simulink model "tfg"  (R2020b)
settings: Solver=VariableStepAuto  StartTime=0.0  StopTime=1  RelTol=1e-3
values from neighbouring files (symbols this model uses):
  k = 0.814    [tfgm.m]
  Kic = R/Tc    (= 500)    [tfgm.m]
  Kpc = L/Tc    (= 5.4)    [tfgm.m]
  P_ = -7000    [tfgm.m]
  Q_ = -5000    [tfgm.m]
undefined symbols (not defined in the file or in its folder): ll, rl
libraries: powerlib x11, pid_lib x2
settings Model: Creator=ssivo  LastModifiedBy=ssivo
settings SolverCC: AlgebraicLoopSolver=LineSearch

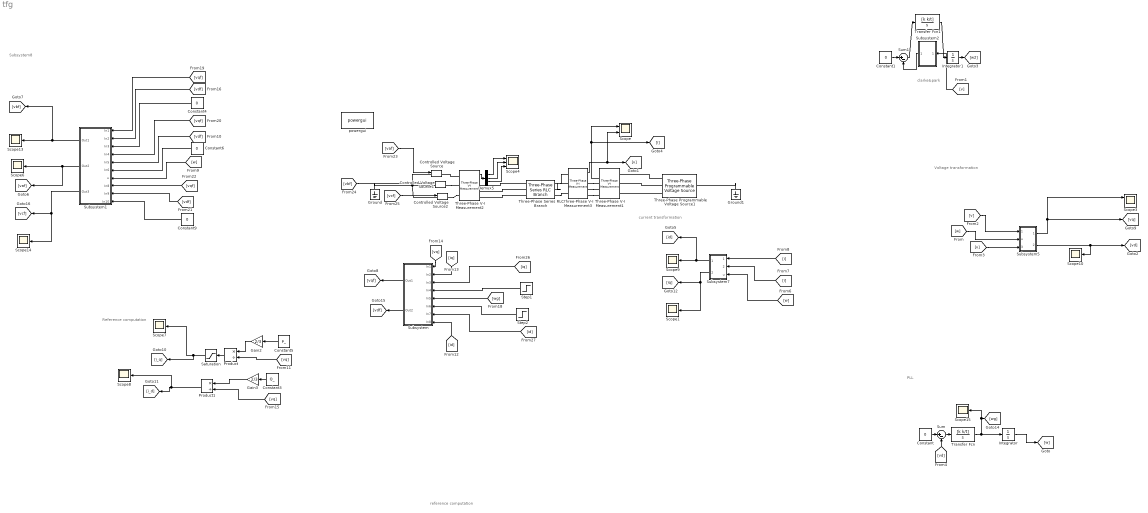
== system tfg ==
  note: Subsystem8
  note: Voltage transformation
  note: PLL
  note: current transformation
  note: Reference computation
  note: reference computation
  note: clarke&park
  Constant{,1,4,6,9} (5 alike) : Constant  Value=0
  Constant3 : Constant  Value=Q_
  Constant5 : Constant  Value=P_
  Controlled Voltage Source : powerlib/Electrical Sources/Controlled Voltage Source  Initialize=on  Source_Type=AC  Amplitude=400  Phase=0  Frequency=50  Measurements=None
  Controlled Voltage Source1 : powerlib/Electrical Sources/Controlled Voltage Source  Initialize=on  Source_Type=AC  Amplitude=400  Phase=0  Frequency=50  Measurements=None
  Controlled Voltage Source2 : powerlib/Electrical Sources/Controlled Voltage Source  Initialize=on  Source_Type=AC  Amplitude=400  Phase=0  Frequency=50  Measurements=None
  Demux5 : Demux  Outputs=3
  Gain2 : Gain  Gain=2/3
  Gain3 : Gain  Gain=2/3
  Ground : powerlib/Elements/Ground  LConnTagsString=a
  Ground1 : powerlib/Elements/Ground  LConnTagsString=a
  Integrator : Integrator
  Integrator1 : Integrator
  Product : Product  Inputs=*/
  Product1 : Product  Inputs=*/
  Saturation : Saturate  UpperLimit=0  LowerLimit=-15
  Scope : Scope  NumInputPorts=2
  Scope{1,6..10,13..15} (9 alike) : Scope
  Scope3 : Scope  NumInputPorts=2
  Scope4 : Scope  NumInputPorts=3
  Step1 : Step  Time=0.2  After=-14.29  SampleTime=0
  Step2 : Step  Time=0.1  After=-10.21  SampleTime=0
  Subsystem : Subsystem
  Subsystem1 : Subsystem
  Subsystem2 : Subsystem
  Subsystem5 : Subsystem
  Subsystem7 : Subsystem
  Sum : Sum  Inputs=|+-
  Sum1 : Sum  Inputs=|+-
  Three-Phase Programmable Voltage Source1 : powerlib/Electrical Sources/Three-Phase Programmable Voltage Source  PositiveSequence="[400  0 50]"  VariationEntity=None  VariationType=Table of time-amplitude pairs  VariationTypeAlt=Step  VariationStep=0.5  VariationRate=10  VariationMagnitude=0.3  VariationFrequency=2  VariationTiming=[1 2]  VariationPhaseA=off  Amplitudes=[1 0.8 1.2 1.0]  TimeValues=[0 0.1 0.15 0.2]  HarmonicGeneration=off  HarmonicA=[3 0.2 -25 0]  HarmonicB=[2 0.15 35 2]  Timing="[0.05  3]"  BusType=swing  Pref=0  Qref=0  Qmin=-inf  Qmax=inf
  Three-Phase Series RLC Branch : powerlib/Elements/Three-Phase Series RLC Branch  LConnTagsString=A|B|C  RConnTagsString=A|B|C  BranchType=RL  Resistance=rl  Inductance=ll  Capacitance=1e-6  Measurements=Branch currents
  Three-Phase V-I Measurement1 : powerlib/Measurements/Three-Phase V-I Measurement  VoltageMeasurement=phase-to-ground  SetLabelV=off  LabelV=Vabc  Vpu=off  VpuLL=off  CurrentMeasurement=yes  SetLabelI=off  LabelI=Iabc  Ipu=off  Pbase=100e6  Vbase=500e3  OutputType=Complex  PhasorSimulation=off  PSBequivalent=0
  Three-Phase V-I Measurement2 : powerlib/Measurements/Three-Phase V-I Measurement  VoltageMeasurement=phase-to-ground  SetLabelV=off  LabelV=Vabc  Vpu=off  VpuLL=off  CurrentMeasurement=yes  SetLabelI=off  LabelI=Iabc  Ipu=off  Pbase=100e6  Vbase=500e3  OutputType=Complex  PhasorSimulation=off  PSBequivalent=0
  Three-Phase V-I Measurement3 : powerlib/Measurements/Three-Phase V-I Measurement  VoltageMeasurement=phase-to-ground  SetLabelV=off  LabelV=Vabc  Vpu=off  VpuLL=off  CurrentMeasurement=yes  SetLabelI=off  LabelI=Iabc  Ipu=off  Pbase=100e6  Vbase=500e3  OutputType=Complex  PhasorSimulation=off  PSBequivalent=0
  Transfer Fcn : TransferFcn  Numerator=[k k/t]  Denominator=[1 0]
  Transfer Fcn1 : TransferFcn  Numerator=[k k/t]  Denominator=[1 0]
  powergui : powerlib/powergui  Priority=1  SimulationMode=Continuous  SampleTime=1e-5  frequency=60  Iterations=50  frequencyindice=50  Pbase=100e6  ErrMax=1e-4  UnitsV=kV  UnitsW=MW  buscounter=0  FunctionMessages=off  echomessages=off  EnableUseOfTLC=off  CurrentSourceSwitches=off  DisableSnubberDevices=off  DisableRonSwitches=off  DisableVfSwitches=off  DisplayEquations=off  AutomaticDiscreteSolvers=off  SolverType=Tustin/Backward Euler (TBE)  Interpol=off  ExternalGateDelay=off  methode=off  Ts=100  x0status=blocks  SPID=on  SwTol=0  HookPort=off  NonlinearTolerance=1e-4  nMaxIteration=100  ContinueOnMaxIteration=off  RestoreLinks=warning  ResistiveCurrentMeasurement=off  Frange=[0:2:500]  Ylog=off  Xlog=on  ShowGrid=off  save=off  variable=ZData  structure=0  ZoomFFT=off  StartTime=0.0  cycles=1  DisplayStyle=1  fundamental=60  FreqAxis=off  MaxFrequency=1000  frequencyindicesteady=1  RmsSteady=1  display=off
  wires:
  Transfer Fcn/1 -> Scope15/1, [wg], Integrator/1
  Constant/1 -> Sum/1
  Sum/1 -> Transfer Fcn/1
  [vd] -> Sum/2
  Sum1/1 -> Transfer Fcn1/1
  Transfer Fcn1/1 -> Integrator1/1
  Constant1/1 -> Sum1/1
  Integrator1/1 -> [w2]
  Subsystem2/1(Out1) -> Sum1/2
  [v] -> Subsystem2/1(In1)
  Three-Phase V-I Measurement1/2 -> [i], Scope/1
  Three-Phase V-I Measurement2/1 -> Demux5/1
  Demux5/1 -> Scope4/1
  Gain3/1 -> Product1/1
  Constant3/1 -> Gain3/1
  [vq] -> Product1/2
  Constant5/1 -> Gain2/1
  [vq] -> Product/2
  Gain2/1 -> Product/1
  Product/1 -> Saturation/1
  Product1/1 -> Scope8/1, [i_d]
  Demux5/2 -> Scope4/2
  Demux5/3 -> Scope4/3
  Integrator/1 -> [w]
  [vaf] -> Controlled Voltage Source/1
  [vbf] -> Controlled Voltage Source1/1
  [vcf] -> Controlled Voltage Source2/1
  Saturation/1 -> [i_q], Scope7/1
  [vq] -> Subsystem/1(In1)
  [iq] -> Subsystem/2(In2)
  [iq] -> Subsystem/3(In3)
  Step1/1 -> Subsystem/4(In4)
  [wg] -> Subsystem/5(In5)
  Step2/1 -> Subsystem/6(In6)
  [id] -> Subsystem/7(In7)
  [id] -> Subsystem/8(In8)
  Subsystem/1(Out1) -> [vqf]
  Subsystem/2(Out2) -> [vdf]
  Subsystem1/2(Out2) -> Scope6/1, [vaf]
  Subsystem1/3(Out3) -> Scope14/1, [vcf]
  Subsystem1/1(Out1) -> [vbf], Scope13/1
  [vqf] -> Subsystem1/1(In1)
  [vdf] -> Subsystem1/2(In2)
  Constant4/1 -> Subsystem1/3(In3)
  [vqf] -> Subsystem1/4(In4)
  [vdf] -> Subsystem1/5(In5)
  Constant6/1 -> Subsystem1/6(In6)
  [w] -> Subsystem1/7(u)
  [vqf] -> Subsystem1/8(In8)
  [vdf] -> Subsystem1/9(In9)
  Constant9/1 -> Subsystem1/10(In10)
  Subsystem7/2(Out2) -> Scope1/1, [iq]
  Subsystem7/1(Out1) -> [id], Scope9/1
  [i] -> Subsystem7/1(In1)
  [i] -> Subsystem7/2(In2)
  [w] -> Subsystem7/3(u)
  Subsystem5/2(Out2) -> Scope10/1, [vd]
  Subsystem5/1(Out1) -> Scope3/1, [vq]
  [v] -> Subsystem5/1(In1)
  [w] -> Subsystem5/2(u)
  [v] -> Subsystem5/3(In3)
  Three-Phase V-I Measurement3/1 -> Scope/2, [v]
  connections:
  Controlled Voltage Source1/RConn1 -- Three-Phase V-I Measurement2/LConn2
  Ground/LConn1 -- Controlled Voltage Source/LConn1 -- Controlled Voltage Source2/LConn1 -- Controlled Voltage Source1/LConn1
  Three-Phase V-I Measurement2/LConn1 -- Controlled Voltage Source/RConn1
  Controlled Voltage Source2/RConn1 -- Three-Phase V-I Measurement2/LConn3
  Three-Phase Programmable Voltage Source1/RConn1 -- Three-Phase V-I Measurement1/LConn1
  Three-Phase Programmable Voltage Source1/RConn2 -- Three-Phase V-I Measurement1/LConn2
  Three-Phase Programmable Voltage Source1/RConn3 -- Three-Phase V-I Measurement1/LConn3
  Ground1/LConn1 -- Three-Phase Programmable Voltage Source1/LConn1
  Three-Phase Series RLC Branch/LConn3 -- Three-Phase V-I Measurement2/RConn3
  Three-Phase Series RLC Branch/LConn2 -- Three-Phase V-I Measurement2/RConn2
  Three-Phase Series RLC Branch/LConn1 -- Three-Phase V-I Measurement2/RConn1
  Three-Phase Series RLC Branch/RConn1 -- Three-Phase V-I Measurement3/LConn1
  Three-Phase Series RLC Branch/RConn2 -- Three-Phase V-I Measurement3/LConn2
  Three-Phase Series RLC Branch/RConn3 -- Three-Phase V-I Measurement3/LConn3
  Three-Phase V-I Measurement3/RConn1 -- Three-Phase V-I Measurement1/RConn1
  Three-Phase V-I Measurement3/RConn2 -- Three-Phase V-I Measurement1/RConn2
  Three-Phase V-I Measurement3/RConn3 -- Three-Phase V-I Measurement1/RConn3

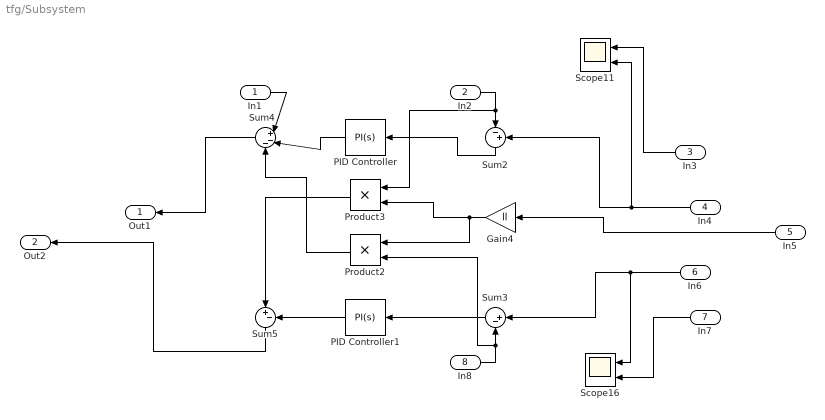
== system tfg/Subsystem ==
  In1 : Inport
  In2 : Inport  Port=2
  In3 : Inport  Port=3
  In4 : Inport  Port=4
  In5 : Inport  Port=5
  In6 : Inport  Port=6
  In7 : Inport  Port=7
  In8 : Inport  Port=8
  Gain4 : Gain  Gain=ll
  PID Controller : pid_lib/PID Controller  Controller=PI  Form=Parallel  TimeDomain=Continuous-time  UseExternalTs=off  SampleTime=-1  IntegratorMethod=Forward Euler  FilterMethod=Forward Euler  ControllerParametersSource=internal  P=Kpc  I=Kic  D=0  UseFilter=on  N=100  TunerSelectOption=Transfer Function Based (PID Tuner App)  InitialConditionSource=internal  InitialConditionForIntegrator=0  InitialConditionForFilter=0  DifferentiatorICPrevScaledInput=0  ExternalReset=none  TrackingMode=off  Kt=1  LimitOutput=off  SatLimitsSource=internal  UpperSaturationLimit=inf  LowerSaturationLimit=-inf  LinearizeAsGain=on  AntiWindupMode=none  Kb=1  POutMin=[]  POutMax=[]  IOutMin=[]  IOutMax=[]  DOutMin=[]  DOutMax=[]  NOutMin=[]  NOutMax=[]  SumOutMin=[]  SumOutMax=[]  SaturationOutMin=[]  SaturationOutMax=[]  PParamMin=[]  PParamMax=[]  IParamMin=[]  IParamMax=[]  DParamMin=[]  DParamMax=[]  NParamMin=[]  NParamMax=[]  KbParamMin=[]  KbParamMax=[]  KtParamMin=[]  KtParamMax=[]  KbOutMin=[]  KbOutMax=[]  KtOutMin=[]  KtOutMax=[]  IntegratorOutMin=[]  IntegratorOutMax=[]  FilterOutMin=[]  FilterOutMax=[]  SumI1OutMin=[]  SumI1OutMax=[]  SumI2OutMin=[]  SumI2OutMax=[]  SumI3OutMin=[]  SumI3OutMax=[]  SumI4OutMin=[]  SumI4OutMax=[]  SumDOutMin=[]  SumDOutMax=[]  DifferentiatorOutMin=[]  DifferentiatorOutMax=[]  FilterDiffOutCoefMin=[]  FilterDiffOutCoefMax=[]  ReciprocalOutMin=[]  ReciprocalOutMax=[]  SumDenOutMin=[]  SumDenOutMax=[]  SumNumOutMin=[]  SumNumOutMax=[]  DivideOutMin=[]  DivideOutMax=[]  UdiffTsProdOutMin=[]  UdiffTsProdOutMax=[]  NTsProdOutMin=[]  NTsProdOutMax=[]  UintegralTsProdOutMin=[]  UintegralTsProdOutMax=[]  UngainTsProdOutMin=[]  UngainTsProdOutMax=[]  IntegratorContinuousStateAttributes=''  IntegratorStateMustResolveToSignalObject=off  IntegratorRTWStateStorageClass=Auto  FilterContinuousStateAttributes=''  FilterStateMustResolveToSignalObject=off  FilterRTWStateStorageClass=Auto  ParallelPVariant=InternalParameters  IdealPVariant=Disabled  IVariant=InternalParameters  DVariant=Disabled  IntegratorVariant=Continuous  SatVariant=Disabled  AWVariant=Passthrough  PCopyVariant=Disabled  TRVariant=Disabled  FdbkBlocksVariant=Forward  IdealPFdbkVariant=Disabled  SatFdbkVariant=Disabled  DerivativeFilterVariant=Disabled  NVariant=Disabled  NCopyVariant=Disabled_SignalSpec  FilterICVariant=Disabled  IntegratorICVariant=InternalICs  ExternalResetVariant=Disabled  TRSumVariant=Passthrough  SumFdbkVariant=Disabled  SumVariant=Sum_PI  TsampFilterVariant=InternalTs  TsampNgainVariant=Passthrough  TsampIntegralVariant=Passthrough  ExternalSaturationOutDataTypeStr=Inherit: Same as second input
  PID Controller1 : pid_lib/PID Controller  Controller=PI  Form=Parallel  TimeDomain=Continuous-time  UseExternalTs=off  SampleTime=-1  IntegratorMethod=Forward Euler  FilterMethod=Forward Euler  ControllerParametersSource=internal  P=Kpc  I=Kic  D=0  UseFilter=on  N=100  TunerSelectOption=Transfer Function Based (PID Tuner App)  InitialConditionSource=internal  InitialConditionForIntegrator=0  InitialConditionForFilter=0  DifferentiatorICPrevScaledInput=0  ExternalReset=none  TrackingMode=off  Kt=1  LimitOutput=off  SatLimitsSource=internal  UpperSaturationLimit=inf  LowerSaturationLimit=-inf  LinearizeAsGain=on  AntiWindupMode=none  Kb=1  POutMin=[]  POutMax=[]  IOutMin=[]  IOutMax=[]  DOutMin=[]  DOutMax=[]  NOutMin=[]  NOutMax=[]  SumOutMin=[]  SumOutMax=[]  SaturationOutMin=[]  SaturationOutMax=[]  PParamMin=[]  PParamMax=[]  IParamMin=[]  IParamMax=[]  DParamMin=[]  DParamMax=[]  NParamMin=[]  NParamMax=[]  KbParamMin=[]  KbParamMax=[]  KtParamMin=[]  KtParamMax=[]  KbOutMin=[]  KbOutMax=[]  KtOutMin=[]  KtOutMax=[]  IntegratorOutMin=[]  IntegratorOutMax=[]  FilterOutMin=[]  FilterOutMax=[]  SumI1OutMin=[]  SumI1OutMax=[]  SumI2OutMin=[]  SumI2OutMax=[]  SumI3OutMin=[]  SumI3OutMax=[]  SumI4OutMin=[]  SumI4OutMax=[]  SumDOutMin=[]  SumDOutMax=[]  DifferentiatorOutMin=[]  DifferentiatorOutMax=[]  FilterDiffOutCoefMin=[]  FilterDiffOutCoefMax=[]  ReciprocalOutMin=[]  ReciprocalOutMax=[]  SumDenOutMin=[]  SumDenOutMax=[]  SumNumOutMin=[]  SumNumOutMax=[]  DivideOutMin=[]  DivideOutMax=[]  UdiffTsProdOutMin=[]  UdiffTsProdOutMax=[]  NTsProdOutMin=[]  NTsProdOutMax=[]  UintegralTsProdOutMin=[]  UintegralTsProdOutMax=[]  UngainTsProdOutMin=[]  UngainTsProdOutMax=[]  IntegratorContinuousStateAttributes=''  IntegratorStateMustResolveToSignalObject=off  IntegratorRTWStateStorageClass=Auto  FilterContinuousStateAttributes=''  FilterStateMustResolveToSignalObject=off  FilterRTWStateStorageClass=Auto  ParallelPVariant=InternalParameters  IdealPVariant=Disabled  IVariant=InternalParameters  DVariant=Disabled  IntegratorVariant=Continuous  SatVariant=Disabled  AWVariant=Passthrough  PCopyVariant=Disabled  TRVariant=Disabled  FdbkBlocksVariant=Forward  IdealPFdbkVariant=Disabled  SatFdbkVariant=Disabled  DerivativeFilterVariant=Disabled  NVariant=Disabled  NCopyVariant=Disabled_SignalSpec  FilterICVariant=Disabled  IntegratorICVariant=InternalICs  ExternalResetVariant=Disabled  TRSumVariant=Passthrough  SumFdbkVariant=Disabled  SumVariant=Sum_PI  TsampFilterVariant=InternalTs  TsampNgainVariant=Passthrough  TsampIntegralVariant=Passthrough  ExternalSaturationOutDataTypeStr=Inherit: Same as second input
  Product2 : Product
  Product3 : Product
  Scope11 : Scope  NumInputPorts=2
  Scope16 : Scope  NumInputPorts=2
  Sum2 : Sum  Inputs=|-+
  Sum3 : Sum  Inputs=|+-
  Sum4 : Sum  Inputs=|+--
  Sum5 : Sum  Inputs=|+-
  Out1 : Outport
  Out2 : Outport  Port=2
  wires:
  Sum2/1 -> PID Controller/1
  In4/1 -> Sum2/2, Scope11/2
  Sum3/1 -> PID Controller1/1
  In6/1 -> Sum3/1, Scope16/1
  PID Controller/1 -> Sum4/2
  Product3/1 -> Sum5/1
  In1/1 -> Sum4/1
  In2/1 -> Product3/1, Sum2/1
  In3/1 -> Scope11/1
  Product2/1 -> Sum4/3
  In8/1 -> Product2/2, Sum3/2
  Gain4/1 -> Product2/1, Product3/2
  PID Controller1/1 -> Sum5/2
  In7/1 -> Scope16/2
  Sum5/1 -> Out2/1
  Sum4/1 -> Out1/1
  In5/1 -> Gain4/1

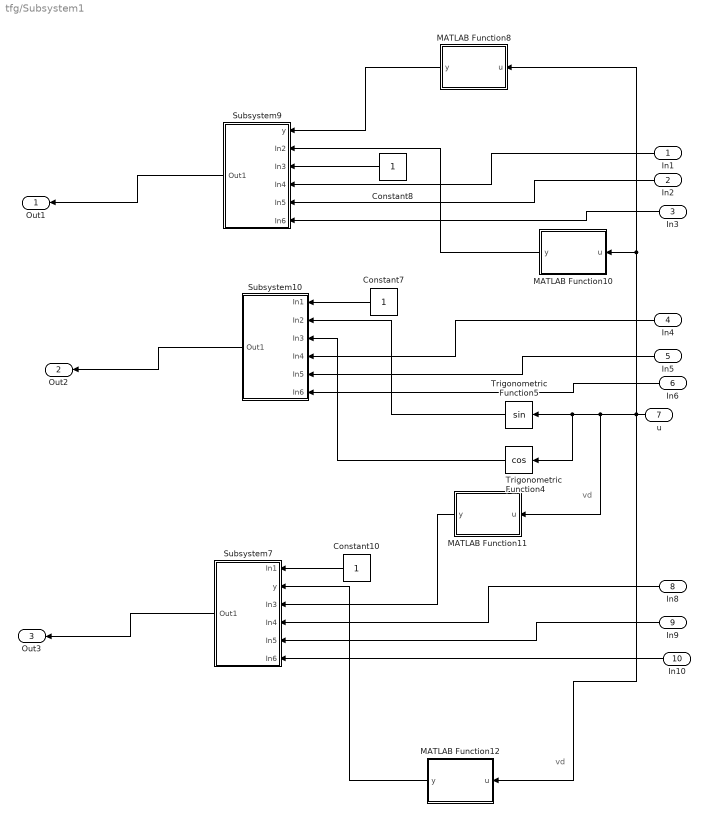
== system tfg/Subsystem1 ==
  note: vd
  note: vd
  In1 : Inport
  In2 : Inport  Port=2
  In3 : Inport  Port=3
  In4 : Inport  Port=4
  In5 : Inport  Port=5
  In6 : Inport  Port=6
  u : Inport  Port=7
  In8 : Inport  Port=8
  In9 : Inport  Port=9
  In10 : Inport  Port=10
  Constant10 : Constant
  Constant7 : Constant
  Constant8 : Constant
  MATLAB Function10 : MATLAB Function  TreatAsAtomicUnit=on
  MATLAB Function11 : MATLAB Function  TreatAsAtomicUnit=on
  MATLAB Function12 : MATLAB Function  TreatAsAtomicUnit=on
  MATLAB Function8 : MATLAB Function  TreatAsAtomicUnit=on
  Subsystem10 : Subsystem
  Subsystem7 : Subsystem
  Subsystem9 : Subsystem
  Trigonometric Function4 : Trigonometry  Operator=cos
  Trigonometric Function5 : Trigonometry
  Out1 : Outport
  Out2 : Outport  Port=2
  Out3 : Outport  Port=3
  wires:
  Trigonometric Function5/1 -> Subsystem10/2(In2)
  MATLAB Function12/1(y) -> Subsystem7/2(y)
  Trigonometric Function4/1 -> Subsystem10/3(In3)
  u/1 -> MATLAB Function12/1(u), MATLAB Function11/1(u), Trigonometric Function4/1, Trigonometric Function5/1, MATLAB Function10/1(u), MATLAB Function8/1(u)
  Subsystem10/1(Out1) -> Out2/1
  Constant10/1 -> Subsystem7/1(In1)
  MATLAB Function8/1(y) -> Subsystem9/1(y)
  Constant8/1 -> Subsystem9/3(In3)
  MATLAB Function11/1(y) -> Subsystem7/3(In3)
  In10/1 -> Subsystem7/6(In6)
  Subsystem7/1(Out1) -> Out3/1
  In8/1 -> Subsystem7/4(In4)
  MATLAB Function10/1(y) -> Subsystem9/2(In2)
  Constant7/1 -> Subsystem10/1(In1)
  In3/1 -> Subsystem9/6(In6)
  In4/1 -> Subsystem10/4(In4)
  In2/1 -> Subsystem9/5(In5)
  In1/1 -> Subsystem9/4(In4)
  In6/1 -> Subsystem10/6(In6)
  In5/1 -> Subsystem10/5(In5)
  In9/1 -> Subsystem7/5(In5)
  Subsystem9/1(Out1) -> Out1/1

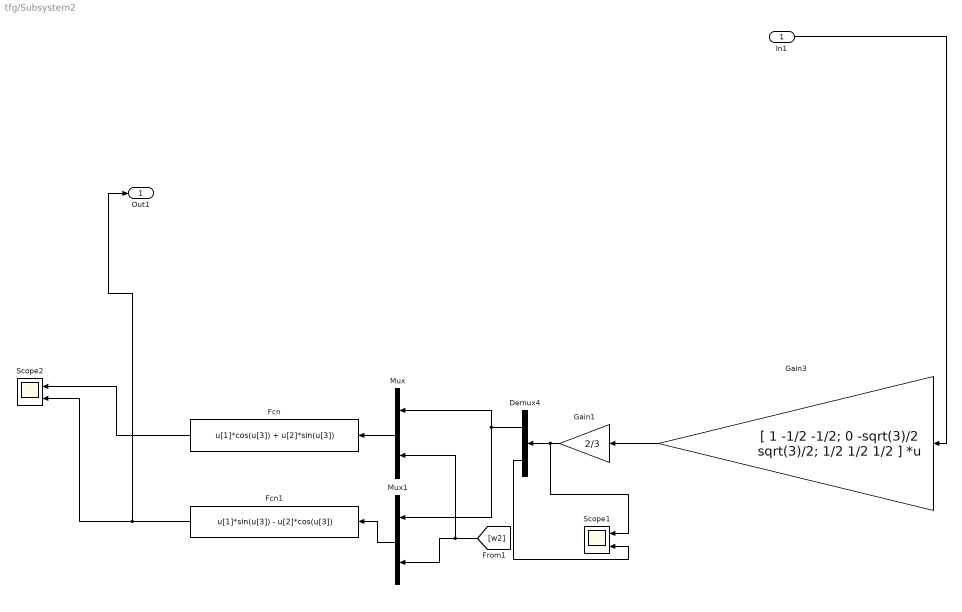
== system tfg/Subsystem2 ==
  In1 : Inport
  Demux4 : Demux  Outputs=[2 1]
  Fcn : Fcn  Expr=u[1]*cos(u[3]) + u[2]*sin(u[3])
  Fcn1 : Fcn  Expr=u[1]*sin(u[3]) - u[2]*cos(u[3])
  Gain1 : Gain  Gain=2/3  SaturateOnIntegerOverflow=on  OutDataTypeStr=Inherit: Same as input  ParamDataTypeStr=Inherit: Same as input
  Gain3 : Gain  Gain="[ 1   -1/2   -1/2; 0   -sqrt(3)/2   sqrt(3)/2; 1/2  1/2  1/2 ]"  Multiplication=Matrix(K*u) (u vector)  SaturateOnIntegerOverflow=on  OutDataTypeStr=Inherit: Same as input  ParamDataTypeStr=Inherit: Same as input
  Mux : Mux  Inputs=2
  Mux1 : Mux  Inputs=2
  Scope1 : Scope  NumInputPorts=2
  Scope2 : Scope  NumInputPorts=2
  Out1 : Outport
  wires:
  Demux4/2 -> Scope1/2
  Fcn/1 -> Scope2/1
  [w2] -> Mux/2, Mux1/2
  Gain3/1 -> Gain1/1
  Mux1/1 -> Fcn1/1
  Gain1/1 -> Scope1/1, Demux4/1
  Mux/1 -> Fcn/1
  Demux4/1 -> Mux1/1, Mux/1
  Fcn1/1 -> Out1/1, Scope2/2
  In1/1 -> Gain3/1

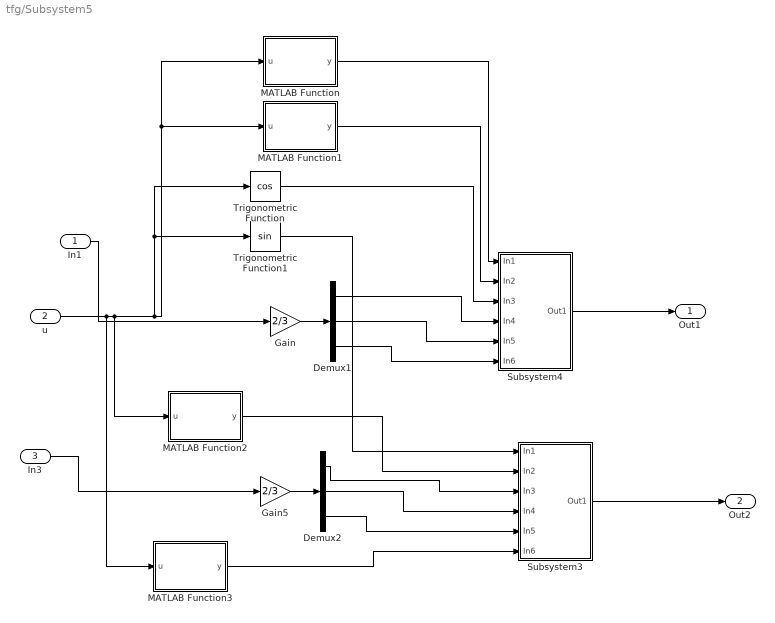
== system tfg/Subsystem5 ==
  In1 : Inport
  u : Inport  Port=2
  In3 : Inport  Port=3
  Demux1 : Demux  Outputs=[1 1 1]
  Demux2 : Demux  Outputs=[1 1 1]
  Gain : Gain  Gain=2/3
  Gain5 : Gain  Gain=2/3
  MATLAB Function : MATLAB Function  TreatAsAtomicUnit=on
  MATLAB Function1 : MATLAB Function  TreatAsAtomicUnit=on
  MATLAB Function2 : MATLAB Function  TreatAsAtomicUnit=on
  MATLAB Function3 : MATLAB Function  TreatAsAtomicUnit=on
  Subsystem3 : Subsystem
  Subsystem4 : Subsystem
  Trigonometric Function : Trigonometry  Operator=cos
  Trigonometric Function1 : Trigonometry
  Out1 : Outport
  Out2 : Outport  Port=2
  wires:
  Trigonometric Function1/1 -> Subsystem3/1(In1)
  Demux1/1 -> Subsystem4/4(In4)
  MATLAB Function3/1(y) -> Subsystem3/6(In6)
  MATLAB Function2/1(y) -> Subsystem3/2(In2)
  Demux1/3 -> Subsystem4/6(In6)
  Demux2/3 -> Subsystem3/5(In5)
  MATLAB Function/1(y) -> Subsystem4/1(In1)
  Demux2/2 -> Subsystem3/4(In4)
  Demux1/2 -> Subsystem4/5(In5)
  Demux2/1 -> Subsystem3/3(In3)
  MATLAB Function1/1(y) -> Subsystem4/2(In2)
  Trigonometric Function/1 -> Subsystem4/3(In3)
  u/1 -> MATLAB Function/1(u), MATLAB Function1/1(u), Trigonometric Function/1, Trigonometric Function1/1, MATLAB Function2/1(u), MATLAB Function3/1(u)
  Subsystem3/1(Out1) -> Out2/1
  Gain5/1 -> Demux2/1
  Gain/1 -> Demux1/1
  In3/1 -> Gain5/1
  In1/1 -> Gain/1
  Subsystem4/1(Out1) -> Out1/1

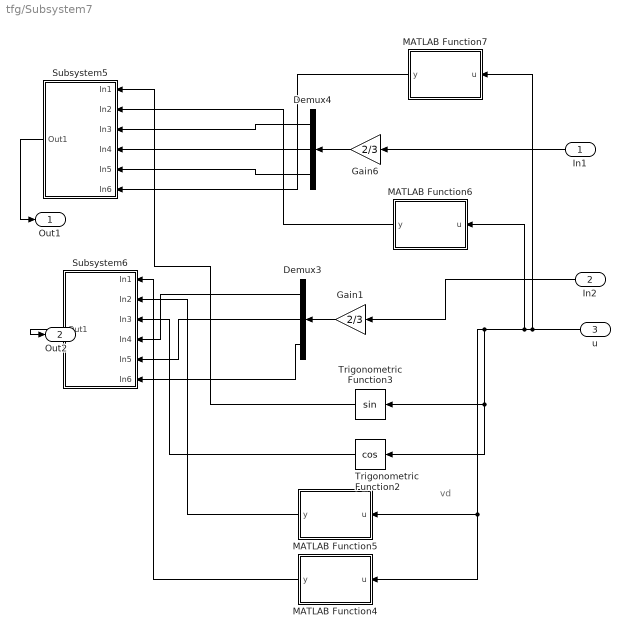
== system tfg/Subsystem7 ==
  note: vd
  In1 : Inport
  In2 : Inport  Port=2
  u : Inport  Port=3
  Demux3 : Demux  Outputs=[1 1 1]
  Demux4 : Demux  Outputs=[1 1 1]
  Gain1 : Gain  Gain=2/3
  Gain6 : Gain  Gain=2/3
  MATLAB Function4 : MATLAB Function  TreatAsAtomicUnit=on
  MATLAB Function5 : MATLAB Function  TreatAsAtomicUnit=on
  MATLAB Function6 : MATLAB Function  TreatAsAtomicUnit=on
  MATLAB Function7 : MATLAB Function  TreatAsAtomicUnit=on
  Subsystem5 : Subsystem
  Subsystem6 : Subsystem
  Trigonometric Function2 : Trigonometry  Operator=cos
  Trigonometric Function3 : Trigonometry
  Out1 : Outport
  Out2 : Outport  Port=2
  wires:
  Demux3/2 -> Subsystem6/5(In5)
  Demux3/1 -> Subsystem6/4(In4)
  Subsystem6/1(Out1) -> Out2/1
  Demux3/3 -> Subsystem6/6(In6)
  Gain1/1 -> Demux3/1
  Gain6/1 -> Demux4/1
  Demux4/3 -> Subsystem5/5(In5)
  MATLAB Function4/1(y) -> Subsystem6/1(In1)
  Trigonometric Function3/1 -> Subsystem5/1(In1)
  Trigonometric Function2/1 -> Subsystem6/3(In3)
  Demux4/1 -> Subsystem5/3(In3)
  MATLAB Function5/1(y) -> Subsystem6/2(In2)
  u/1 -> Trigonometric Function2/1, Trigonometric Function3/1, MATLAB Function5/1(u), MATLAB Function4/1(u), MATLAB Function6/1(u), MATLAB Function7/1(u)
  Demux4/2 -> Subsystem5/4(In4)
  MATLAB Function7/1(y) -> Subsystem5/6(In6)
  MATLAB Function6/1(y) -> Subsystem5/2(In2)
  In2/1 -> Gain1/1
  In1/1 -> Gain6/1
  Subsystem5/1(Out1) -> Out1/1

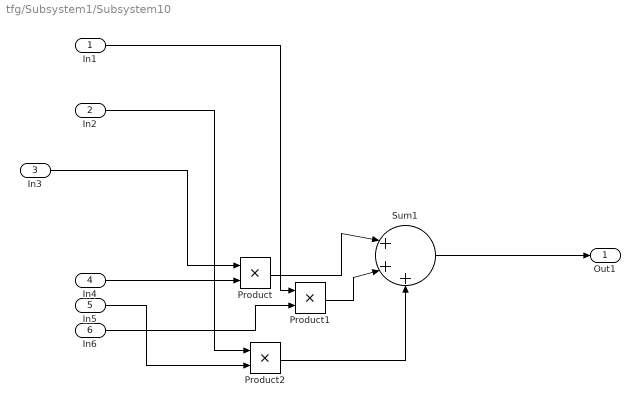
== system tfg/Subsystem1/Subsystem10 ==
  In1 : Inport
  In2 : Inport  Port=2
  In3 : Inport  Port=3
  In4 : Inport  Port=4
  In5 : Inport  Port=5
  In6 : Inport  Port=6
  Product : Product
  Product1 : Product
  Product2 : Product
  Sum1 : Sum  Inputs=|+++
  Out1 : Outport
  wires:
  Product1/1 -> Sum1/2
  In2/1 -> Product2/1
  Product2/1 -> Sum1/3
  In3/1 -> Product/1
  In5/1 -> Product2/2
  Product/1 -> Sum1/1
  In6/1 -> Product1/2
  In1/1 -> Product1/1
  In4/1 -> Product/2
  Sum1/1 -> Out1/1

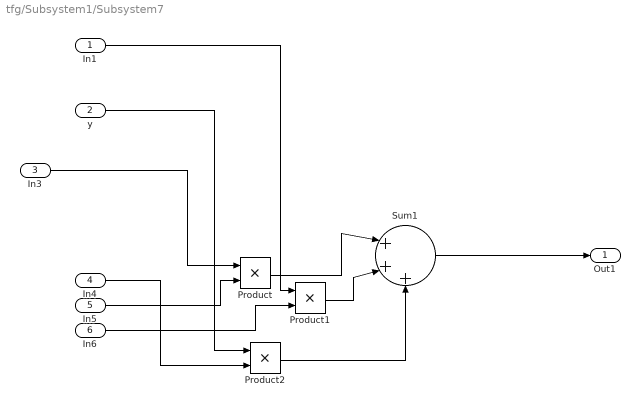
== system tfg/Subsystem1/Subsystem7 ==
  In1 : Inport
  y : Inport  Port=2
  In3 : Inport  Port=3
  In4 : Inport  Port=4
  In5 : Inport  Port=5
  In6 : Inport  Port=6
  Product : Product
  Product1 : Product
  Product2 : Product
  Sum1 : Sum  Inputs=|+++
  Out1 : Outport
  wires:
  Product1/1 -> Sum1/2
  y/1 -> Product2/1
  Product2/1 -> Sum1/3
  In3/1 -> Product/1
  In5/1 -> Product/2
  Product/1 -> Sum1/1
  In6/1 -> Product1/2
  In1/1 -> Product1/1
  In4/1 -> Product2/2
  Sum1/1 -> Out1/1

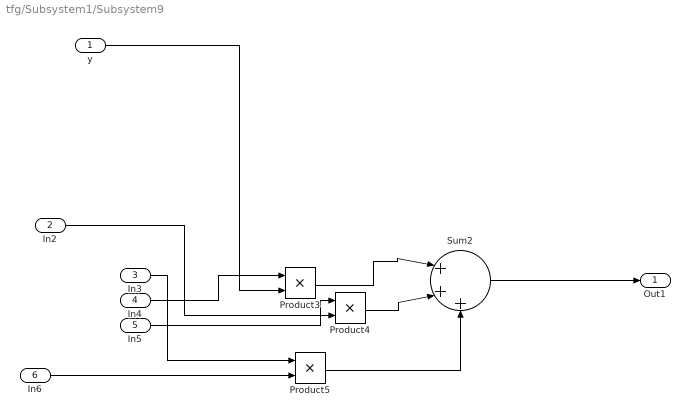
== system tfg/Subsystem1/Subsystem9 ==
  y : Inport
  In2 : Inport  Port=2
  In3 : Inport  Port=3
  In4 : Inport  Port=4
  In5 : Inport  Port=5
  In6 : Inport  Port=6
  Product3 : Product
  Product4 : Product
  Product5 : Product
  Sum2 : Sum  Inputs=|+++
  Out1 : Outport
  wires:
  In4/1 -> Product3/1
  In6/1 -> Product5/2
  Product3/1 -> Sum2/1
  Product4/1 -> Sum2/2
  In5/1 -> Product4/1
  Product5/1 -> Sum2/3
  In3/1 -> Product5/1
  y/1 -> Product3/2
  In2/1 -> Product4/2
  Sum2/1 -> Out1/1

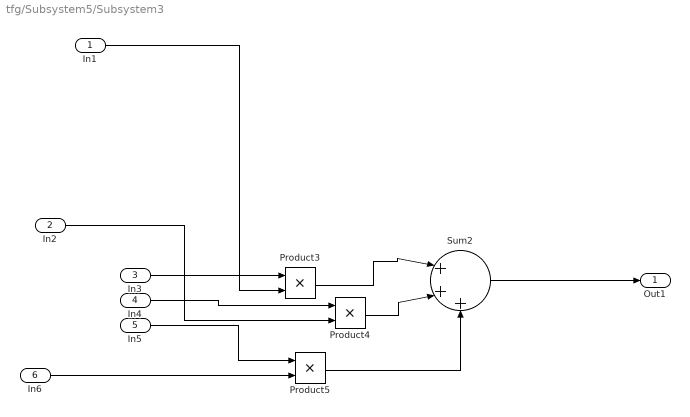
== system tfg/Subsystem5/Subsystem3 ==
  In1 : Inport
  In2 : Inport  Port=2
  In3 : Inport  Port=3
  In4 : Inport  Port=4
  In5 : Inport  Port=5
  In6 : Inport  Port=6
  Product3 : Product
  Product4 : Product
  Product5 : Product
  Sum2 : Sum  Inputs=|+++
  Out1 : Outport
  wires:
  In4/1 -> Product4/1
  In6/1 -> Product5/2
  Product3/1 -> Sum2/1
  Product4/1 -> Sum2/2
  In5/1 -> Product5/1
  Product5/1 -> Sum2/3
  In3/1 -> Product3/1
  In1/1 -> Product3/2
  In2/1 -> Product4/2
  Sum2/1 -> Out1/1

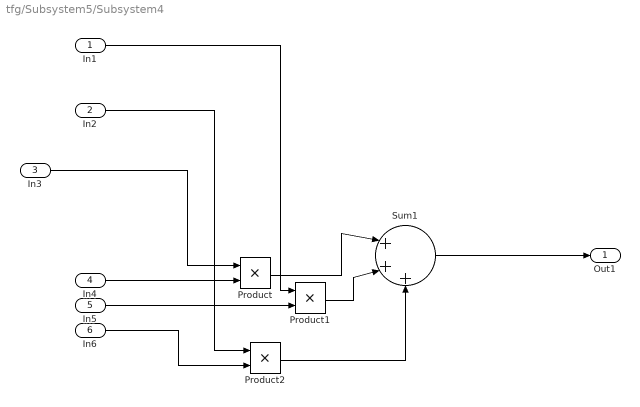
== system tfg/Subsystem5/Subsystem4 ==
  In1 : Inport
  In2 : Inport  Port=2
  In3 : Inport  Port=3
  In4 : Inport  Port=4
  In5 : Inport  Port=5
  In6 : Inport  Port=6
  Product : Product
  Product1 : Product
  Product2 : Product
  Sum1 : Sum  Inputs=|+++
  Out1 : Outport
  wires:
  Product1/1 -> Sum1/2
  In2/1 -> Product2/1
  Product2/1 -> Sum1/3
  In3/1 -> Product/1
  In5/1 -> Product1/2
  Product/1 -> Sum1/1
  In6/1 -> Product2/2
  In1/1 -> Product1/1
  In4/1 -> Product/2
  Sum1/1 -> Out1/1

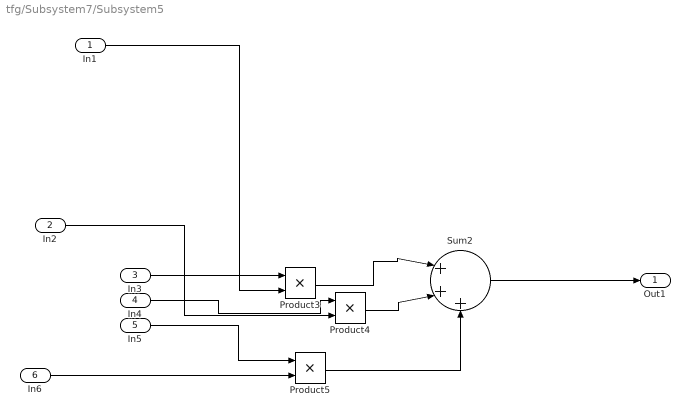
== system tfg/Subsystem7/Subsystem5 ==
  In1 : Inport
  In2 : Inport  Port=2
  In3 : Inport  Port=3
  In4 : Inport  Port=4
  In5 : Inport  Port=5
  In6 : Inport  Port=6
  Product3 : Product
  Product4 : Product
  Product5 : Product
  Sum2 : Sum  Inputs=|+++
  Out1 : Outport
  wires:
  In4/1 -> Product4/1
  In6/1 -> Product5/2
  Product3/1 -> Sum2/1
  Product4/1 -> Sum2/2
  In5/1 -> Product5/1
  Product5/1 -> Sum2/3
  In3/1 -> Product3/1
  In1/1 -> Product3/2
  In2/1 -> Product4/2
  Sum2/1 -> Out1/1

== system tfg/Subsystem7/Subsystem6 ==
  In1 : Inport
  In2 : Inport  Port=2
  In3 : Inport  Port=3
  In4 : Inport  Port=4
  In5 : Inport  Port=5
  In6 : Inport  Port=6
  Product : Product
  Product1 : Product
  Product2 : Product
  Sum1 : Sum  Inputs=|+++
  Out1 : Outport
  wires:
  Product1/1 -> Sum1/2
  In2/1 -> Product2/1
  Product2/1 -> Sum1/3
  In3/1 -> Product/1
  In5/1 -> Product1/2
  Product/1 -> Sum1/1
  In6/1 -> Product2/2
  In1/1 -> Product1/1
  In4/1 -> Product/2
  Sum1/1 -> Out1/1

== matlab function tfg/Subsystem5/MATLAB Function ==
  data: u input; y output
function y = fcn(u)

y = cos(u-2*pi/3);

== matlab function tfg/Subsystem5/MATLAB Function2 ==
  data: u input; y output
function y = fcn(u)

y = sin(u-2*pi/3);

== matlab function tfg/Subsystem5/MATLAB Function3 ==
  data: u input; y output
function y = fcn(u)

y = sin(u+2*pi/3);

== matlab function tfg/Subsystem7/MATLAB Function4 ==
  data: u input; y output
function y = fcn(u)

y = cos(u-2*pi/3);

== matlab function tfg/Subsystem7/MATLAB Function5 ==
  data: u input; y output
function y = fcn(u)

y = cos(u+2*pi/3);

== matlab function tfg/Subsystem7/MATLAB Function6 ==
  data: u input; y output
function y = fcn(u)

y = sin(u-2*pi/3);

== matlab function tfg/Subsystem7/MATLAB Function7 ==
  data: u input; y output
function y = fcn(u)

y = sin(u+2*pi/3);

== matlab function tfg/Subsystem1/MATLAB Function10 ==
  data: u input; y output
function y = fcn(u)

y = sin(u-2*pi/3);

== matlab function tfg/Subsystem5/MATLAB Function1 ==
  data: u input; y output
function y = fcn(u)

y = cos(u+2*pi/3);

== matlab function tfg/Subsystem1/MATLAB Function11 ==
  data: u input; y output
function y = fcn(u)

y = sin(u+2*pi/3);

== matlab function tfg/Subsystem1/MATLAB Function8 ==
  data: u input; y output
function y = fcn(u)

y = cos(u-2*pi/3);

== matlab function tfg/Subsystem1/MATLAB Function12 ==
  data: u input; y output
function y = fcn(u)

y = cos(u+2*pi/3);
